simulink model "MPC_project"  (R2024b)
settings: Solver=VariableStepAuto  StartTime=0.0  StopTime=10.0  RelTol=1e-3
undefined symbols (not defined in the file or in its folder): Discrete, Time
libraries: ctrlSharedLib x1, mpclib x1
settings Model: Creator=galax  LastModifiedBy=galax
settings DebuggingCC: UnderSpecifiedDimensionMsg=warning

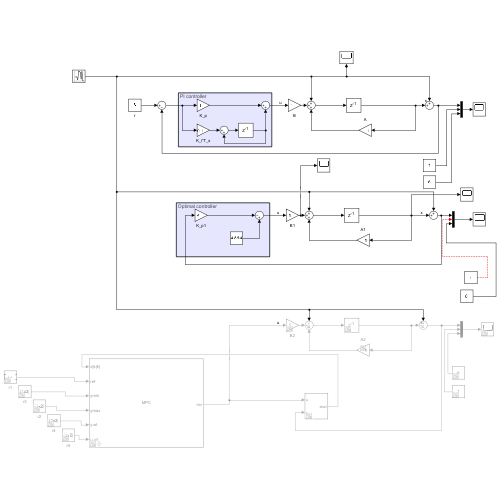
[thumbnail: Simulink's stored preview of the top-level diagram]
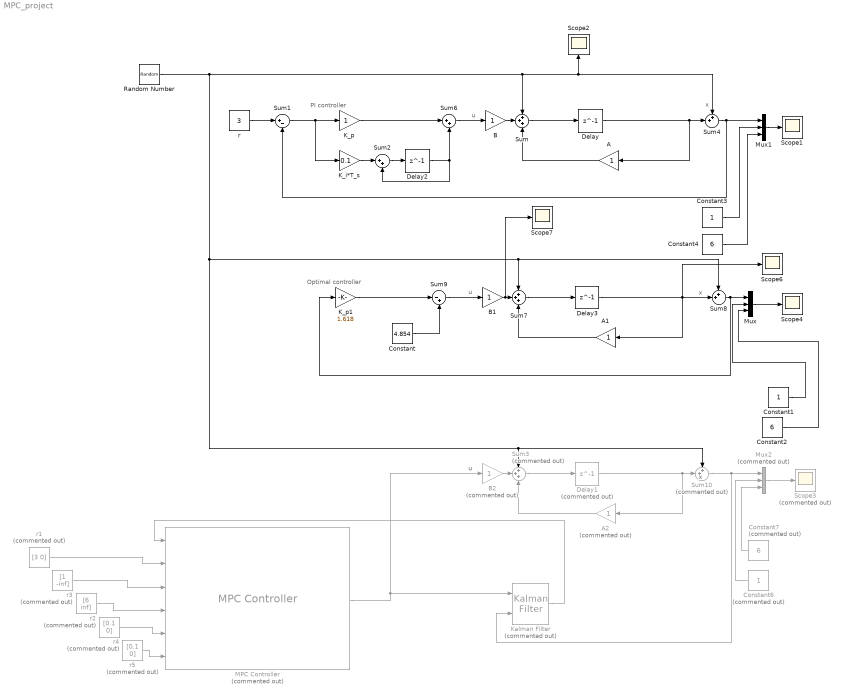
== system MPC_project ==
  note: PI controller
  note: x
  note: u
  note: u
  note: x
  note: Optimal controller
  note: u
  note: x
  A : Gain
  A1 : Gain
  A2 : Gain  Commented=on
  B : Gain
  B1 : Gain
  B2 : Gain  Commented=on
  Constant : Constant  Value=4.854
  Constant1 : Constant
  Constant2 : Constant  Value=6
  Constant3 : Constant
  Constant4 : Constant  Value=6
  Constant6 : Constant  Commented=on
  Constant7 : Constant  Commented=on  Value=6
  Delay : Delay  DelayLength=1  InitialCondition=2  SampleTime=0.1
  Delay1 : Delay  Commented=on  DelayLength=1  InitialCondition=2  SampleTime=0.1
  Delay2 : Delay  DelayLength=1  InitialCondition=0  SampleTime=0.1
  Delay3 : Delay  DelayLength=1  InitialCondition=2  SampleTime=0.1
  K_i*T_s : Gain  Gain=0.1
  K_p : Gain
  K_p1 : Gain  Gain=1.618
  Kalman Filter : ctrlSharedLib/Kalman Filter  Commented=on  TimeDomain=Discrete-Time  UseCurrentEstimator=on  ModelSource=Individual A, B, C, D matrices  ModelSourceVariable=ss(0.95,1,1,0,1)  A=1  B=1  C=1  D=0  NumberOfStates=1  NumberOfInputs=1  NumberOfOutputs=1  InitialEstimateSource=Dialog  X0=2  P0=10  UseK=off  UseGH=off  NumberOfProcessNoiseInputs=1  G=1  TimeInvariantG=on  H=0  TimeInvariantH=on  Q=0.1  TimeInvariantQ=on  R=0.1  TimeInvariantR=on  N=0  TimeInvariantN=on  AddInputPort=on  AddEnablePort=off  OutputEstimatedY=off  OutputP=off  Ts=-1
  MPC Controller : mpclib/MPC Controller  Commented=on  SCDEnableBlockLinearizationSpecification=on  is_multiple=0  enable_value=0  return_u0=off  updateMPCinCallerWorkspace=on  md_inport=off  mv_inport=off  uref_inport=off  return_cost=off  return_mvseq=off  return_qpstatus=off  return_xseq=off  return_state=off  return_ovseq=off  state_inport=on  umin_inport=off  umax_inport=off  ymin_inport=on  ymax_inport=on  cc_inport=off  ywt_inport=on  uwt_inport=on  duwt_inport=off  rhoeps_inport=off  pm_inport=off  MaximumP=100  HorizonChoice=FixedHorizon  n_ts=0.1  n_p=100  n_mv=1  n_md=1  n_ud=1  n_mo=1  n_uo=0  BlockDataType=double  SampleTimeInherited=off  switch_inport=off
  Mux : Mux  Inputs=3
  Mux1 : Mux  Inputs=3
  Mux2 : Mux  Commented=on  Inputs=3
  Random Number : RandomNumber  Variance=0.1  SampleTime=0.1
  Scope{1..2,4,6..7} (5 alike) : Scope
  Scope3 : Scope  Commented=on
  Sum : Sum  Inputs=+++
  Sum1 : Sum  Inputs=|+-
  Sum10 : Sum  Commented=on  Inputs=++|
  Sum2 : Sum  Inputs=|++
  Sum3 : Sum  Commented=on  Inputs=+++
  Sum4 : Sum  Inputs=++|
  Sum6 : Sum  Inputs=|++
  Sum7 : Sum  Inputs=+++
  Sum8 : Sum  Inputs=++|
  Sum9 : Sum  Inputs=|-+
  r : Constant  Value=3
  r1 : Constant  Commented=on  Value=[3 0]
  r2 : Constant  Commented=on  Value=[6 inf]
  r3 : Constant  Commented=on  Value=[1 -inf]
  r4 : Constant  Commented=on  Value=[0.1 0]
  r5 : Constant  Commented=on  Value=[0.1 0]
  wires:
  A/1 -> Sum/3
  Sum/1 -> Delay/1
  r/1 -> Sum1/1
  B/1 -> Sum/2
  Sum1/1 -> K_i*T_s/1, K_p/1
  K_i*T_s/1 -> Sum2/1
  Sum2/1 -> Delay2/1
  Delay2/1 -> Sum6/2, Sum2/2
  Sum6/1 -> B/1
  K_p/1 -> Sum6/1
  B1/1 -> Scope7/1, Sum7/2
  Delay3/1 -> Scope6/1, A1/1, Sum8/2
  Sum7/1 -> Delay3/1
  K_p1/1 -> Sum9/1
  A1/1 -> Sum7/3
  Sum9/1 -> B1/1
  Constant/1 -> Sum9/2
  Constant1/1 -> Mux/2
  Constant2/1 -> Mux/3
  Mux/1 -> Scope4/1
  Constant4/1 -> Mux1/3
  Constant3/1 -> Mux1/2
  Delay/1 -> Sum4/2, A/1
  Mux1/1 -> Scope1/1
  B2/1 -> Sum3/2
  A2/1 -> Sum3/3
  MPC Controller/1 -> B2/1, Kalman Filter/1
  Sum3/1 -> Delay1/1
  Delay1/1 -> Sum10/2, A2/1
  Constant7/1 -> Mux2/3
  Constant6/1 -> Mux2/2
  Mux2/1 -> Scope3/1
  Random Number/1 -> Sum4/1, Scope2/1, Sum/1, Sum10/1, Sum3/1, Sum7/1, Sum8/1
  Kalman Filter/1 -> MPC Controller/1
  Sum4/1 -> Sum1/2, Mux1/1
  Sum8/1 -> K_p1/1, Mux/1
  Sum10/1 -> Kalman Filter/2, Mux2/1
  r1/1 -> MPC Controller/2
  r3/1 -> MPC Controller/3
  r2/1 -> MPC Controller/4
  r4/1 -> MPC Controller/5
  r5/1 -> MPC Controller/6
